simulink model "time_response_slx1"  (R2020b)
settings: Solver=VariableStepAuto  StartTime=0.0  StopTime=10.0  RelTol=1e-3
values from neighbouring files (symbols this model uses):
  a = 4    [part0102_reals.m]    (also in part0102_reals_m1.m; part0103_imags_m1.m; part0104_nat_freqs.m; part0104_nat_freqs_m1.m)
  b = 25    [part0102_reals.m]    (also in part0102_reals_m1.m; part0103_imags_m1.m; part0104_nat_freqs.m; part0104_nat_freqs_m1.m)
  G_a = pad    [part03_params_m1.m]
  G_b = pad    [part03_params_m1.m]
settings Model: Creator=Leo Duran  LastModifiedBy=Leo Duran

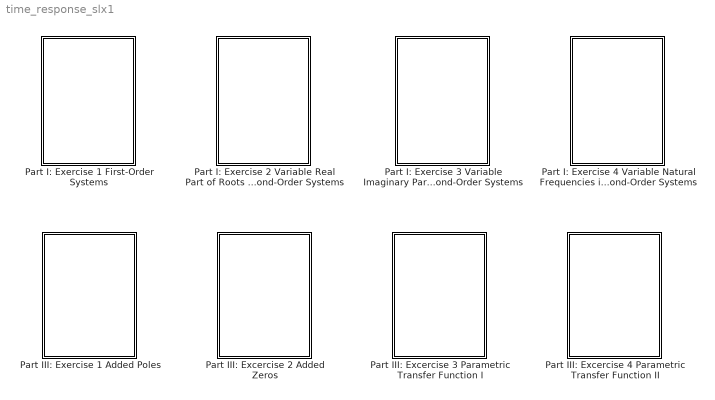
== system time_response_slx1 ==
  Part I: Exercise 1 First-Order Systems : Subsystem
  Part I: Exercise 2 Variable Real Part of Roots in Second-Order Systems : Subsystem
  Part I: Exercise 3 Variable Imaginary Part of Roots in Second-Order Systems : Subsystem
  Part I: Exercise 4 Variable Natural Frequencies in Second-Order Systems : Subsystem
  Part III: Excercise 2 Added Zeros : Subsystem
  Part III: Excercise 3 Parametric Transfer Function I : Subsystem
  Part III: Excercise 4 Parametric Transfer Function II : Subsystem
  Part III: Exercise 1 Added Poles : Subsystem

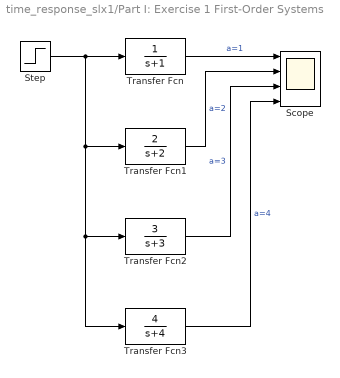
== system time_response_slx1/Part I: Exercise 1 First-Order Systems ==
  Scope : Scope  NumInputPorts=4
  Step : Step  Time=0  SampleTime=0
  Transfer Fcn : TransferFcn  Denominator=[1 1]
  Transfer Fcn1 : TransferFcn  Numerator=[2]  Denominator=[1 2]
  Transfer Fcn2 : TransferFcn  Numerator=[3]  Denominator=[1 3]
  Transfer Fcn3 : TransferFcn  Numerator=[4]  Denominator=[1 4]
  wires:
  Transfer Fcn/1 -> Scope/1  "a=1"
  Step/1 -> Transfer Fcn3/1, Transfer Fcn2/1, Transfer Fcn1/1, Transfer Fcn/1
  Transfer Fcn2/1 -> Scope/3  "a=3"
  Transfer Fcn1/1 -> Scope/2  "a=2"
  Transfer Fcn3/1 -> Scope/4  "a=4"

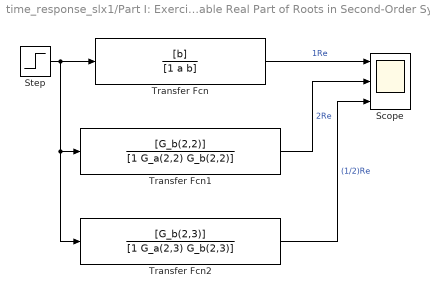
== system time_response_slx1/Part I: Exercise 2 Variable Real Part of Roots in Second-Order Systems ==
  Scope : Scope  NumInputPorts=3
  Step : Step  Time=0  SampleTime=0
  Transfer Fcn : TransferFcn  Numerator=[b]  Denominator=[1 a b]
  Transfer Fcn1 : TransferFcn  Numerator=[G_b(2,2)]  Denominator=[1 G_a(2,2) G_b(2,2)]
  Transfer Fcn2 : TransferFcn  Numerator=[G_b(2,3)]  Denominator=[1 G_a(2,3) G_b(2,3)]
  wires:
  Step/1 -> Transfer Fcn2/1, Transfer Fcn1/1, Transfer Fcn/1
  Transfer Fcn/1 -> Scope/1  "1Re"
  Transfer Fcn2/1 -> Scope/3  "(1/2)Re"
  Transfer Fcn1/1 -> Scope/2  "2Re"

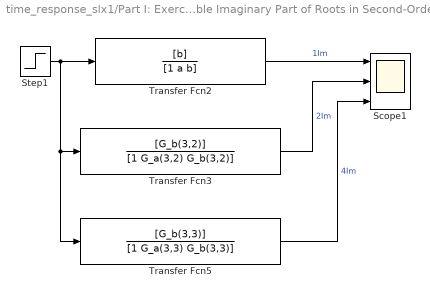
== system time_response_slx1/Part I: Exercise 3 Variable Imaginary Part of Roots in Second-Order Systems ==
  Scope1 : Scope  NumInputPorts=3
  Step1 : Step  Time=0  SampleTime=0
  Transfer Fcn2 : TransferFcn  Numerator=[b]  Denominator=[1 a b]
  Transfer Fcn3 : TransferFcn  Numerator=[G_b(3,2)]  Denominator=[1 G_a(3,2) G_b(3,2)]
  Transfer Fcn5 : TransferFcn  Numerator=[G_b(3,3)]  Denominator=[1 G_a(3,3) G_b(3,3)]
  wires:
  Step1/1 -> Transfer Fcn5/1, Transfer Fcn3/1, Transfer Fcn2/1
  Transfer Fcn5/1 -> Scope1/3  "4Im"
  Transfer Fcn2/1 -> Scope1/1  "1Im"
  Transfer Fcn3/1 -> Scope1/2  "2Im"

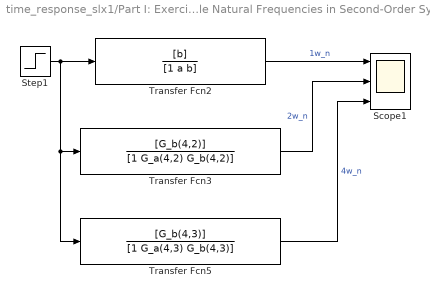
== system time_response_slx1/Part I: Exercise 4 Variable Natural Frequencies in Second-Order Systems ==
  Scope1 : Scope  NumInputPorts=3
  Step1 : Step  Time=0  SampleTime=0
  Transfer Fcn2 : TransferFcn  Numerator=[b]  Denominator=[1 a b]
  Transfer Fcn3 : TransferFcn  Numerator=[G_b(4,2)]  Denominator=[1 G_a(4,2) G_b(4,2)]
  Transfer Fcn5 : TransferFcn  Numerator=[G_b(4,3)]  Denominator=[1 G_a(4,3) G_b(4,3)]
  wires:
  Transfer Fcn2/1 -> Scope1/1  "1w_n"
  Step1/1 -> Transfer Fcn5/1, Transfer Fcn3/1, Transfer Fcn2/1
  Transfer Fcn5/1 -> Scope1/3  "4w_n"
  Transfer Fcn3/1 -> Scope1/2  "2w_n"

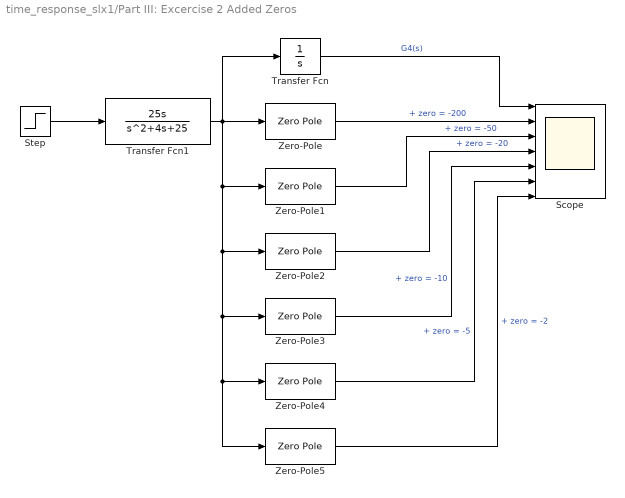
== system time_response_slx1/Part III: Excercise 2 Added Zeros ==
  Scope : Scope  NumInputPorts=7
  Step : Step  Time=0  SampleTime=0
  Transfer Fcn : TransferFcn  Denominator=[1 0]
  Transfer Fcn1 : TransferFcn  Numerator=[25 0]  Denominator=[1 4 25]
  Zero-Pole : ZeroPole  Zeros=[-200]  Poles=[0]
  Zero-Pole1 : ZeroPole  Zeros=[-50]  Poles=[0]
  Zero-Pole2 : ZeroPole  Zeros=[-20]  Poles=[0]
  Zero-Pole3 : ZeroPole  Zeros=[-10]  Poles=[0]
  Zero-Pole4 : ZeroPole  Zeros=[-5]  Poles=[0]
  Zero-Pole5 : ZeroPole  Zeros=[-2]  Poles=[0]
  wires:
  Transfer Fcn1/1 -> Zero-Pole/1, Transfer Fcn/1, Zero-Pole1/1, Zero-Pole2/1, Zero-Pole3/1, Zero-Pole5/1, Zero-Pole4/1
  Step/1 -> Transfer Fcn1/1
  Zero-Pole/1 -> Scope/2  "+ zero = -200"
  Zero-Pole1/1 -> Scope/3  "+ zero = -50"
  Zero-Pole2/1 -> Scope/4  "+ zero = -20"
  Zero-Pole3/1 -> Scope/5  "+ zero = -10"
  Zero-Pole4/1 -> Scope/6  "+ zero = -5"
  Zero-Pole5/1 -> Scope/7  "+ zero = -2"
  Transfer Fcn/1 -> Scope/1  "G4(s)"

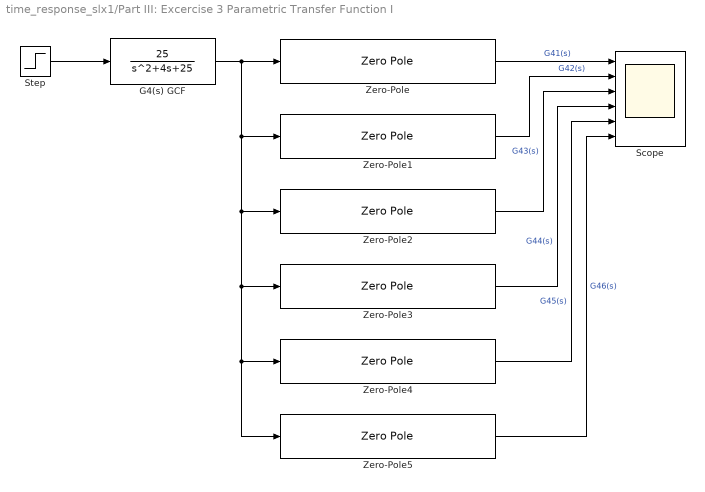
== system time_response_slx1/Part III: Excercise 3 Parametric Transfer Function I ==
  G4(s) GCF : TransferFcn  Numerator=[25]  Denominator=[1 4 25]
  Scope : Scope  NumInputPorts=6
  Step : Step  Time=0  SampleTime=0
  Zero-Pole : ZeroPole  Zeros=[-G_a(7,1)]  Poles=[-G_b(7,1)]  Gain=G_b(7,1)/G_a(7,1)
  Zero-Pole1 : ZeroPole  Zeros=[-G_a(7,2)]  Poles=[-G_b(7,2)]  Gain=G_b(7,2)/G_a(7,2)
  Zero-Pole2 : ZeroPole  Zeros=[-G_a(7,3)]  Poles=[-G_b(7,3)]  Gain=G_b(7,3)/G_a(7,3)
  Zero-Pole3 : ZeroPole  Zeros=[-G_a(7,4)]  Poles=[-G_b(7,4)]  Gain=G_b(7,4)/G_a(7,4)
  Zero-Pole4 : ZeroPole  Zeros=[-G_a(7,5)]  Poles=[-G_b(7,5)]  Gain=G_b(7,5)/G_a(7,5)
  Zero-Pole5 : ZeroPole  Zeros=[-G_a(7,6)]  Poles=[-G_b(7,6)]  Gain=G_b(7,6)/G_a(7,6)
  wires:
  Step/1 -> G4(s) GCF/1
  G4(s) GCF/1 -> Zero-Pole5/1, Zero-Pole4/1, Zero-Pole3/1, Zero-Pole2/1, Zero-Pole1/1, Zero-Pole/1
  Zero-Pole/1 -> Scope/1  "G41(s)"
  Zero-Pole1/1 -> Scope/2  "G42(s)"
  Zero-Pole2/1 -> Scope/3  "G43(s)"
  Zero-Pole3/1 -> Scope/4  "G44(s)"
  Zero-Pole4/1 -> Scope/5  "G45(s)"
  Zero-Pole5/1 -> Scope/6  "G46(s)"

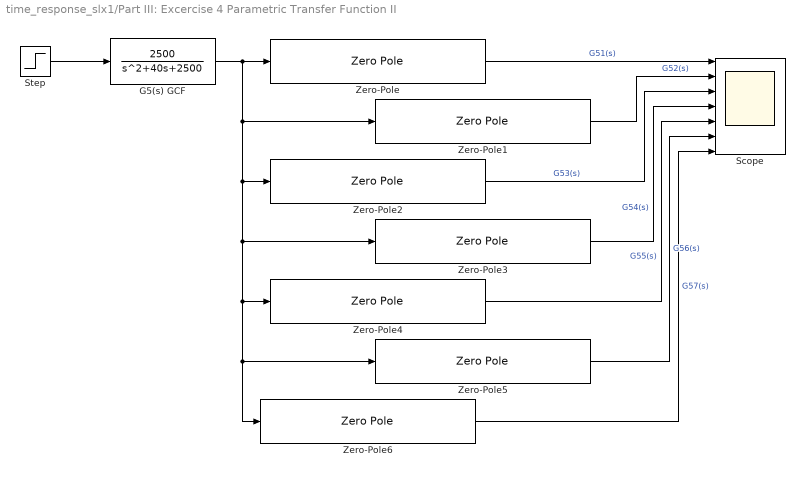
== system time_response_slx1/Part III: Excercise 4 Parametric Transfer Function II ==
  G5(s) GCF : TransferFcn  Numerator=[2500]  Denominator=[1 40 2500]
  Scope : Scope  NumInputPorts=7
  Step : Step  Time=0  SampleTime=0
  Zero-Pole : ZeroPole  Zeros=[-G_a(8,1)]  Poles=[-G_b(8,1)]  Gain=G_b(8,1)/G_a(8,1)
  Zero-Pole1 : ZeroPole  Zeros=[-G_a(8,2)]  Poles=[-G_b(8,2)]  Gain=G_b(8,2)/G_a(8,2)
  Zero-Pole2 : ZeroPole  Zeros=[-G_a(8,3)]  Poles=[-G_b(8,3)]  Gain=G_b(8,3)/G_a(8,3)
  Zero-Pole3 : ZeroPole  Zeros=[-G_a(8,4)]  Poles=[-G_b(8,4)]  Gain=G_b(8,4)/G_a(8,4)
  Zero-Pole4 : ZeroPole  Zeros=[-G_a(8,5)]  Poles=[-G_b(8,5)]  Gain=G_b(8,5)/G_a(8,5)
  Zero-Pole5 : ZeroPole  Zeros=[-G_a(8,6)]  Poles=[-G_b(8,6)]  Gain=G_b(8,6)/G_a(8,6)
  Zero-Pole6 : ZeroPole  Zeros=[-G_a(8,5)]  Poles=[-G_b(8,5)]  Gain=G_b(8,5)/G_a(8,5)
  wires:
  Step/1 -> G5(s) GCF/1
  G5(s) GCF/1 -> Zero-Pole/1, Zero-Pole1/1, Zero-Pole2/1, Zero-Pole3/1, Zero-Pole4/1, Zero-Pole6/1, Zero-Pole5/1
  Zero-Pole/1 -> Scope/1  "G51(s)"
  Zero-Pole1/1 -> Scope/2  "G52(s)"
  Zero-Pole2/1 -> Scope/3  "G53(s)"
  Zero-Pole3/1 -> Scope/4  "G54(s)"
  Zero-Pole4/1 -> Scope/5  "G55(s)"
  Zero-Pole5/1 -> Scope/6  "G56(s)"
  Zero-Pole6/1 -> Scope/7  "G57(s)"

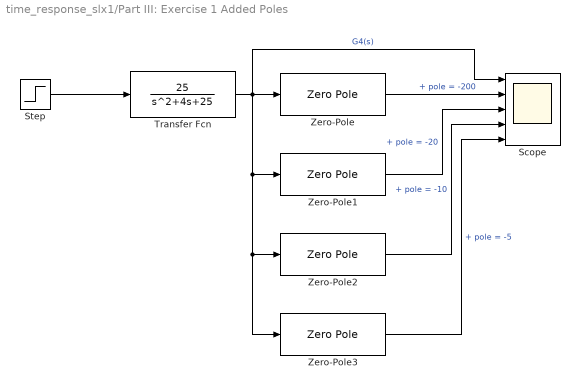
== system time_response_slx1/Part III: Exercise 1 Added Poles ==
  Scope : Scope  NumInputPorts=5
  Step : Step  Time=0  SampleTime=0
  Transfer Fcn : TransferFcn  Numerator=[25]  Denominator=[1 4 25]
  Zero-Pole : ZeroPole  Zeros=[]  Poles=[-200]
  Zero-Pole1 : ZeroPole  Zeros=[]  Poles=[-20]
  Zero-Pole2 : ZeroPole  Zeros=[]  Poles=[-10]
  Zero-Pole3 : ZeroPole  Zeros=[]  Poles=[-5]
  wires:
  Transfer Fcn/1 -> Scope/1, Zero-Pole3/1, Zero-Pole2/1, Zero-Pole1/1, Zero-Pole/1  "G4(s)"
  Step/1 -> Transfer Fcn/1
  Zero-Pole/1 -> Scope/2  "+ pole = -200"
  Zero-Pole1/1 -> Scope/3  "+ pole = -20"
  Zero-Pole2/1 -> Scope/4  "+ pole = -10"
  Zero-Pole3/1 -> Scope/5  "+ pole = -5"
